simulink model "tutorial_vms"  (R2023a)
settings: Solver=FixedStepAuto  StartTime=0.0  StopTime=50  FixedStep=framePeriod_s  RelTol=1e-3
undefined symbols (not defined in the file): Aircraft, framePeriod_s
settings Model: Creator=brian  LastModifiedBy=tuan
settings SolverCC: AlgebraicLoopSolver=TrustRegion
settings OptimizationCC: DefaultParameterBehavior=Inlined  GainParamInheritBuiltInType=on  UseFloatMulNetSlope=on  DefaultUnderspecifiedDataType=single  EnhancedBackFolding=on  BooleansAsBitfields=on  PassReuseOutputArgsAs=Individual arguments  StateBitsets=on  DataBitsets=on  ActiveStateOutputEnumStorageType=uint16  ZeroExternalMemoryAtStartup=off  ZeroInternalMemoryAtStartup=off  EfficientFloat2IntCast=on  LifeSpan=inf  DifferentSizesBufferReuse=on  OptimizationPriority=RAM  OptimizationCustomize=off  EfficientTunableParamExpr=on
settings DebuggingCC: ParameterPrecisionLossMsg=none  ParameterTunabilityLossMsg=error  UnconnectedInputMsg=warning  UnconnectedOutputMsg=warning  UnconnectedLineMsg=warning  BusObjectLabelMismatch=error  RootOutportRequireBusObject=error  NonBusSignalsTreatedAsBus=error  SFInvalidInputDataAccessInChartInitDiag=error  SFTransitionOutsideNaturalParentDiag=error  SFUnreachableExecutionPathDiag=error  SFUndirectedBroadcastEventsDiag=error
settings HardwareCC: ProdBitPerPointer=32  ProdBitPerSizeT=32  ProdBitPerPtrDiffT=32  ProdLargestAtomicInteger=Long  ProdLargestAtomicFloat=Double  ProdWordSize=32  ProdHWDeviceType=NXP->Cortex-M4  TargetLargestAtomicInteger=Long  TargetLargestAtomicFloat=Double  TargetLongLongMode=on  TargetIntDivRoundTo=Zero  TargetEndianess=LittleEndian  TargetHWDeviceType=NXP->Cortex-M4  ProdEqTarget=off
settings ModelReferenceCC: EnableRefExpFcnMdlSchedulingChecks=on  ModelReferenceNumInstancesAllowed=Single
settings SFSimCC: SimParseCustomCode=off  SimGenImportedTypeDefs=on  MATLABDynamicMemAlloc=off  SimTargetLang=C++
settings SFSimCC: SimUserIncludeDirs=|
  | ../../flight_code/include
  | ../../../ua_spaaro_extra/imu/include
  | ../../../ua_spaaro_extra/gnss/include
  | ../../../ua_spaaro_extra/pres/include
  | ../../../ua_spaaro_extra/sbus/include
  | ../../../ua_spaaro_extra/global_defs/include
settings SFSimCC: SimUserDefines=|
  | SIL
  | __FMU_R_MINI_V1__
settings RTWCC: Description=Embedded Coder  SystemTargetFile=ert.tlc  GenCodeOnly=on  TemplateMakefile=ert_default_tmf  GenerateReport=on  RTWVerbose=off  RTWUseSimCustomCode=on  Toolchain=GNU gcc/g++ | gmake (64-bit Linux)  BuildConfiguration=Specify  IncludeHyperlinkInReport=on  LaunchReport=on  TargetLang=C++  GenerateTraceInfo=on  GenerateTraceReport=on  GenerateTraceReportSl=on  GenerateTraceReportSf=on  GenerateTraceReportEml=on  GenerateCodeReplacementReport=on  DLArmComputeVersion=19.05
settings RTWCC: CustomInclude=|
  | ../../flight_code/include
  | ../../../ua_spaaro_extra/imu/include
  | ../../../ua_spaaro_extra/gnss/include
  | ../../../ua_spaaro_extra/pres/include
  | ../../../ua_spaaro_extra/sbus/include
  | ../../../ua_spaaro_extra/global_defs/include
settings RTWCC: CustomDefine=|
  | SIL
  | __FMU_R_MINI_V1__
settings CodeAppCC: ForceParamTrailComments=on  IgnoreCustomStorageClasses=off  OperatorAnnotations=on  SimulinkDataObjDesc=on  SFDataObjDesc=on  MATLABFcnDesc=on  CustomSymbolStrGlobalVar=rt$N$M  CustomSymbolStrType=$N$M  CustomSymbolStrFcn=$N$M$F  CustomSymbolStrMacro=$N$M  InsertBlockDesc=on  StateflowObjectComments=on  MATLABSourceComments=on  EnableCustomComments=on  InternalIdentifier=Classic  InlinedPrmAccess=Macros  ReqsInCode=on
settings ERTTargetCC: TargetLangStandard=C++03 (ISO)  GenerateFullHeader=off  IncludeMdlTerminateFcn=off  CombineSignalStateStructs=on  SuppressErrorStatus=on  SupportAbsoluteTime=off  CodeInterfacePackaging=C++ class  SupportNonFinite=off  SupportComplex=off  ParenthesesLevel=Standards  CastingMode=Standards  ERTHeaderFileRootName=autocode$E  ERTSourceFileRootName=autocode$E  InlinedParameterPlacement=NonHierarchical  RootIOFormat=Structure reference  ERTCustomFileTemplate=example_file_process.tlc  ERTFilePackagingFormat=Compact  PreserveExpressionOrder=on  PreserveIfCondition=on  ConvertIfToSwitch=off  EnableSignedLeftShifts=off  EnableSignedRightShifts=off  IndentSize=4

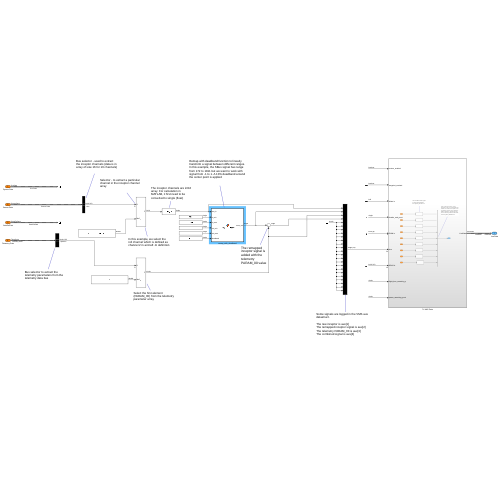
[thumbnail: Simulink's stored preview of the top-level diagram]
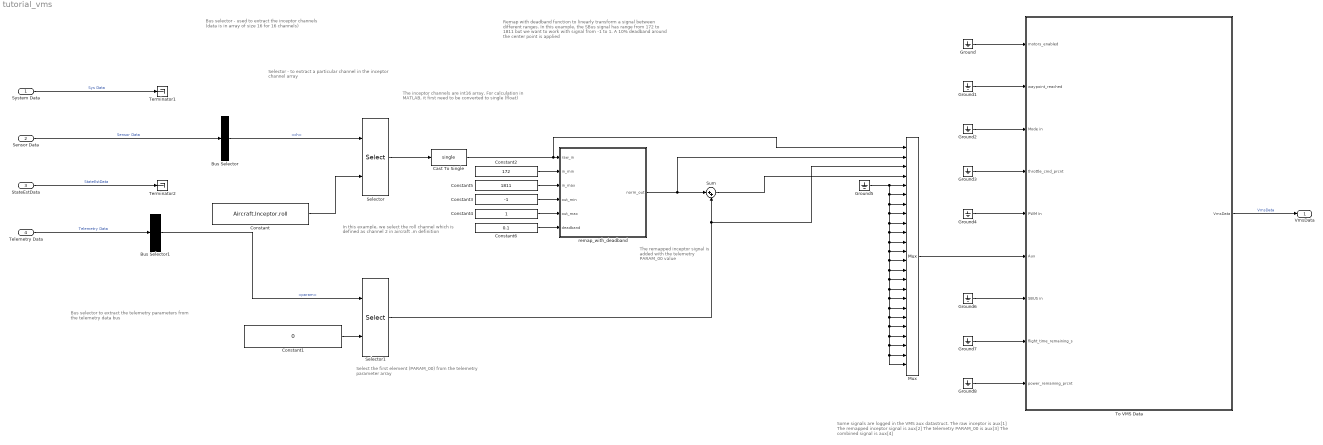
== system tutorial_vms ==
  note: The remapped inceptor signal is added with the telemetry PARAM_00 value
  note: Remap with deadband function to linearly transform a signal between different ranges. In this example, the SBus signal has range from 172 to 1811 but we want to work with signal from -1 to 1. A 10% deadband around the center point is applied
  note: Bus selector - used to extract the inceptor channels (data is in array of size 16 for 16 channels)
  note: Selector - to extract a particular channel in the inceptor channel array
  note: In this example, we select the roll channel which is defined as channel 2 in aircraft .m definition
  note: Select the first element (PARAM_00) from the telemetry parameter array
  note: Bus selector to extract the telemetry parameters from the telemetry data bus
  note: Some signals are logged in the VMS aux datastruct.
      |
      | The raw inceptor is aux[1]
      | The remapped inceptor signal is aux[2]
      | The telemetry PARAM_00 is aux[3]
      | The combined signal is aux[4]
  note: The inceptor channels are int16 array. For calculation in MATLAB, it first need to be converted to single (float)
  System Data : Inport  OutDataTypeStr=Bus: SysData  SampleTime=framePeriod_s  BusOutputAsStruct=on
  Sensor Data : Inport  Port=2  OutDataTypeStr=Bus: SensorData  SampleTime=framePeriod_s  BusOutputAsStruct=on
  StateEstData : Inport  Port=3  OutDataTypeStr=Bus: StateEstData  SampleTime=framePeriod_s  BusOutputAsStruct=on
  Telemetry Data : Inport  Port=4  OutDataTypeStr=Bus: TelemData  SampleTime=framePeriod_s  BusOutputAsStruct=on
  Bus Selector : BusSelector  OutputSignals=inceptor.ch
  Bus Selector1 : BusSelector  OutputSignals=param
  Cast To Single : DataTypeConversion  OutDataTypeStr=single  SaturateOnIntegerOverflow=off  RndMeth=Floor
  Constant : Constant  Value=Aircraft.Inceptor.roll
  Constant1 : Constant  Value=0
  Constant2 : Constant  Value=172  OutDataTypeStr=single
  Constant3 : Constant  Value=-1  OutDataTypeStr=single
  Constant4 : Constant  OutDataTypeStr=single
  Constant5 : Constant  Value=1811  OutDataTypeStr=single
  Constant6 : Constant  Value=0.1  OutDataTypeStr=single
  Ground{,1..8} (9 alike) : Ground
  Mux : Mux  Inputs=24
  Selector : Selector  InputPortWidth=16  IndexOptions=Index vector (port)  Indices=[1 3]  OutputSizes=1
  Selector1 : Selector  IndexMode=Zero-based  InputPortWidth=24  IndexOptions=Index vector (port)  Indices=[1 3]  OutputSizes=1  RuntimeRangeChecks=on
  Sum : Sum  Inputs=|++
  Terminator1 : Terminator
  Terminator2 : Terminator
  To VMS Data : Subsystem
  remap_with_deadband : MATLAB Function  TreatAsAtomicUnit=on
  VmsData : Outport  OutDataTypeStr=Bus: VmsData  SampleTime=framePeriod_s  BusOutputAsStruct=on
  wires:
  To VMS Data/1(VmsData) -> VmsData/1  "VmsData"
  System Data/1 -> Terminator1/1  "Sys Data"
  Sensor Data/1 -> Bus Selector/1  "Sensor Data"
  StateEstData/1 -> Terminator2/1  "StateEstData"
  Telemetry Data/1 -> Bus Selector1/1  "Telemetry Data"
  Ground/1 -> To VMS Data/1(motors_enabled)
  Ground1/1 -> To VMS Data/2(waypoint_reached)
  Ground2/1 -> To VMS Data/3(Mode in)
  Ground3/1 -> To VMS Data/4(throttle_cmd_prcnt)
  Ground4/1 -> To VMS Data/5(PWM In)
  Mux/1 -> To VMS Data/6(Aux)
  Ground6/1 -> To VMS Data/7(SBUS in)
  Ground7/1 -> To VMS Data/8(flight_time_remaining_s)
  Ground8/1 -> To VMS Data/9(power_remaining_prcnt)
  Bus Selector/1 -> Selector/1  "<ch>"
  Constant/1 -> Selector/2
  Bus Selector1/1 -> Selector1/1  "<param>"
  Constant1/1 -> Selector1/2
  Selector/1 -> Cast To Single/1
  Constant2/1 -> remap_with_deadband/2(in_min)
  Constant5/1 -> remap_with_deadband/3(in_max)
  Constant3/1 -> remap_with_deadband/4(out_min)
  Constant4/1 -> remap_with_deadband/5(out_max)
  Constant6/1 -> remap_with_deadband/6(deadband)
  remap_with_deadband/1(norm_out) -> Sum/1, Mux/2
  Selector1/1 -> Mux/3, Sum/2
  Sum/1 -> Mux/4
  Ground5/1 -> Mux/24, Mux/23, Mux/22, Mux/21, Mux/20, Mux/19, Mux/18, Mux/17, Mux/16, Mux/15, Mux/14, Mux/13, Mux/12, Mux/11, Mux/10, Mux/9, Mux/8, Mux/7, Mux/6, Mux/5
  Cast To Single/1 -> Mux/1, remap_with_deadband/1(raw_in)

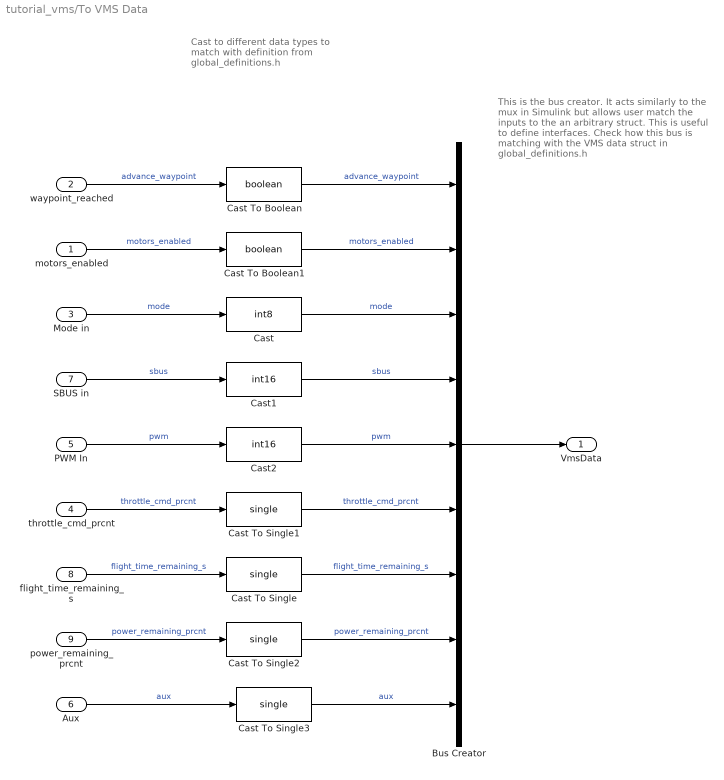
== system tutorial_vms/To VMS Data ==
  note: Cast to different data types to match with definition from global_definitions.h
  note: This is the bus creator. It acts similarly to the mux in Simulink but allows user match the inputs to the an arbitrary struct. This is useful to define interfaces. Check how this bus is matching with the VMS data struct in global_definitions.h
  motors_enabled : Inport
  waypoint_reached : Inport  Port=2
  Mode in : Inport  Port=3
  throttle_cmd_prcnt : Inport  Port=4
  PWM In : Inport  Port=5
  Aux : Inport  Port=6
  SBUS in : Inport  Port=7
  flight_time_remaining_s : Inport  Port=8
  power_remaining_prcnt : Inport  Port=9
  Bus Creator : BusCreator  Inputs=9  OutDataTypeStr=Bus: VmsData  NonVirtualBus=on
      settings: InheritFromInputs=off
  Cast : DataTypeConversion  OutDataTypeStr=int8  SaturateOnIntegerOverflow=off  RndMeth=Floor
  Cast To Boolean : DataTypeConversion  OutDataTypeStr=boolean  SaturateOnIntegerOverflow=off  RndMeth=Floor
  Cast To Boolean1 : DataTypeConversion  OutDataTypeStr=boolean  SaturateOnIntegerOverflow=off  RndMeth=Floor
  Cast To Single{,1..3} (4 alike) : DataTypeConversion  OutDataTypeStr=single  SaturateOnIntegerOverflow=off  RndMeth=Floor
  Cast1 : DataTypeConversion  OutDataTypeStr=int16  SaturateOnIntegerOverflow=off  RndMeth=Floor
  Cast2 : DataTypeConversion  OutDataTypeStr=int16  SaturateOnIntegerOverflow=off  RndMeth=Floor
  VmsData : Outport
  wires:
  Bus Creator/1 -> VmsData/1
  waypoint_reached/1 -> Cast To Boolean/1  "advance_waypoint"
  motors_enabled/1 -> Cast To Boolean1/1  "motors_enabled"
  Mode in/1 -> Cast/1  "mode"
  SBUS in/1 -> Cast1/1  "sbus"
  PWM In/1 -> Cast2/1  "pwm"
  throttle_cmd_prcnt/1 -> Cast To Single1/1  "throttle_cmd_prcnt"
  Aux/1 -> Cast To Single3/1  "aux"
  Cast To Single2/1 -> Bus Creator/8  "power_remaining_prcnt"
  Cast To Single/1 -> Bus Creator/7  "flight_time_remaining_s"
  flight_time_remaining_s/1 -> Cast To Single/1  "flight_time_remaining_s"
  Cast To Boolean/1 -> Bus Creator/1  "advance_waypoint"
  Cast To Boolean1/1 -> Bus Creator/2  "motors_enabled"
  Cast/1 -> Bus Creator/3  "mode"
  Cast1/1 -> Bus Creator/4  "sbus"
  Cast2/1 -> Bus Creator/5  "pwm"
  Cast To Single1/1 -> Bus Creator/6  "throttle_cmd_prcnt"
  power_remaining_prcnt/1 -> Cast To Single2/1  "power_remaining_prcnt"
  Cast To Single3/1 -> Bus Creator/9  "aux"

== matlab function tutorial_vms/remap_with_deadband ==
  data: raw_in input; norm_out output; in_min input; in_max input; out_min input; out_max input; deadband input
function norm_out = remap_deadband(raw_in, in_min, in_max, out_min, out_max, deadband)
in_avg = (in_min + in_max) / 2;
out_avg = (out_min + out_max) / 2;

in_deadband_range = (in_max - in_min) * deadband / 2;
in_deadband_low = in_avg - in_deadband_range;
in_deadband_hi = in_avg + in_deadband_range;

if raw_in < in_deadband_low
    norm_out = (raw_in - in_deadband_low) .* (out_max - out_avg)./(in_deadband_low - in_min) + out_avg;
elseif raw_in > in_deadband_low && raw_in < in_deadband_hi
    norm_out = out_avg;
else
    norm_out = (raw_in - in_deadband_hi) .* (out_max - out_avg)./(in_max - in_deadband_hi) + out_avg;
end
